simulink model "Bandpass_Filter"  (R2014b)
settings: Solver=ode3  StartTime=0.0  StopTime=1  FixedStep=1/5000000  RelTol=1e-3
undefined symbols (not defined in the file or in its folder): dfilt, fdesignblkfcn, gcbh
libraries: dsparch4 x1
settings Model: Creator=Eitima  LastModifiedBy=Eitima
settings DataIOCC: ExternalInput=[t, SigTime]  LimitDataPoints=off  LoadExternalInput=on  TimeSaveName=tOut  OutputSaveName=SigTimeOut

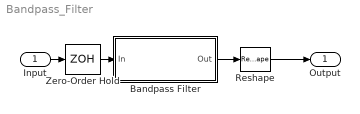
== system Bandpass_Filter ==
  Input : Inport
  Bandpass Filter : Subsystem  DialogController=fdesignblkfcn  InitFcn=fdesignblkfcn(gcbh, {'InitFcn'});  mask(Bandpass Filter){}
      mask help: Design a bandpass filter
      settings: CopyFcn=fdesignblkfcn(gcbh, {'CopyFcn'});
      mask Help: helpview(mapfilelocation('dsp'), 'dspbandpassfilter');
      mask Display: disp('Bandpass');
  Reshape : Reshape
  Zero-Order Hold : ZeroOrderHold  SampleTime=-1
  Output : Outport
  wires:
  Reshape/1 -> Output/1
  Bandpass Filter/1(Out) -> Reshape/1
  Input/1 -> Zero-Order Hold/1
  Zero-Order Hold/1 -> Bandpass Filter/1(In)

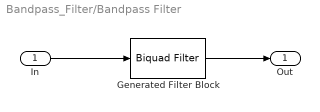
== system Bandpass_Filter/Bandpass Filter ==
  In : Inport
  Generated Filter Block : dsparch4/Biquad Filter  Tag=BlockMethodSubSystem  IIRFiltStruct=Direct form II  CoeffSource=Specify via dialog  BiQuadCoeffs=[0.01013958648634297 0 -0.01013958648634297 1 -1.6618133812024951 0.98627046054740486;0.0025493781187891492 0 -0.0025493781187891492 1 -1.6514591991218408 0.98607730419032968;0.016304485317952876 0 -0.016304485317952876 1 -1.6744504392878072 0.99677925049276372;0.010019474414157988 0 -0.010019474414157988 1 -1.6562936076737262 0.99669840495107032;0.011567698875754661 0 -0.011567698875754661 1 -1.6564338939134684 0.98375080085450683;0.0047790385123797378 0 -0.0047790385123797378 1 -1.6527923586273903 0.98367098468879577;0.014421092390225715 0 -0.014421092390225715 1 -1.6681267322604891 0.99083770350510236;0.91340939446196634 0 -0.91340939446196634 1 -1.6526752268318703 0.99064368018868598]  a0Flag=Warning  IC=0  ICnum=0  ICden=0  InputProcessing=Columns as channels (frame based)  denAccumFracLength=30  denProdOutputFracLength=30  secondMemoryFracLength=15  roundingMode=Floor  overflowMode=off  ScaleValues=[0.0075209697231768506;1;1;1;1;1;1;1;1]  optimizeScaleValues=off  ScaleValueMode=Specify via input port (g)  scaleValueFracLength=14  FilterSource=Specify via dialog  dfiltObjectName=dfilt.df2tsos([1 0.3 0.4],[1 0.1 0.2])
  Out : Outport
  wires:
  In/1 -> Generated Filter Block/1
  Generated Filter Block/1 -> Out/1
